simulink model "integer_add_subtract"  (Simulink 7.5)
settings: Solver=ode45  StartTime=0.0  StopTime=10.0  RelTol=1e-3
libraries: xbsIndex_r4 x91
settings Model: Creator=andryc  LastModifiedBy=Murtaza
settings DebuggingCC: StrictBusMsg=Warning

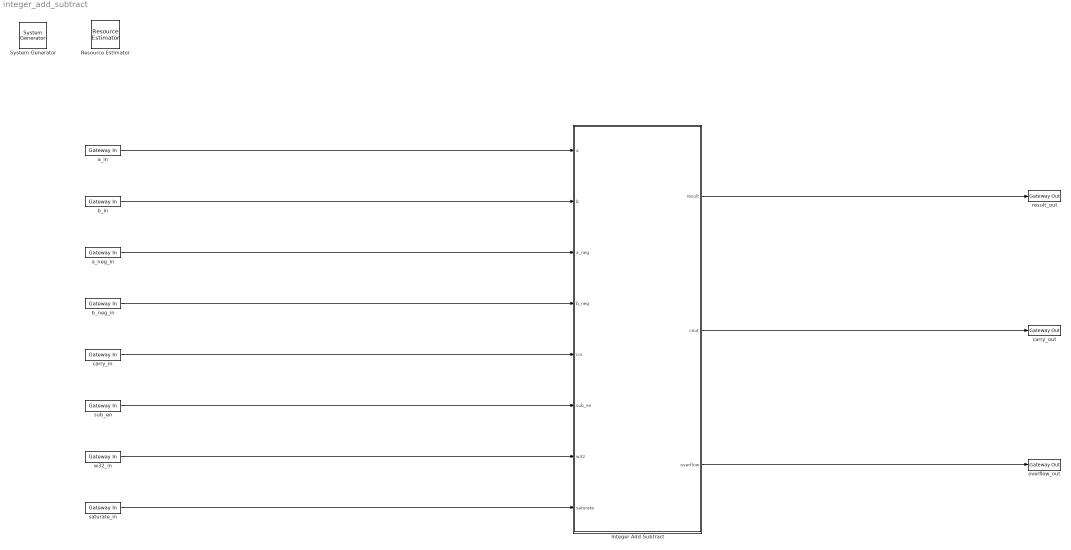
== system integer_add_subtract ==
  " System Generator" : xbsIndex_r4/ System Generator  Tag=genX  SystemSampleTime=-1  xilinxfamily=virtex5  part=xc5vlx330t  speed=-1  package=ff1738  synthesis_tool=XST  clock_wrapper=Clock Enables  directory=./ngc_netlist  proj_type=Project Navigator  testbench=off  simulink_period=1  sysclk_period=3.333333333  dcm_input_clock_period=10  incr_netlist=off  trim_vbits=Everywhere in SubSystem  dbl_ovrd=According to Block Masks  core_generation=According to Block Masks  run_coregen=off  deprecated_control=off  eval_field=0  block_type=sysgen
  Integer Add Subtract : Subsystem
  Resource Estimator : xbsIndex_r4/Resource Estimator  Tag=resEstTag  Slices=0  FFs=0  BRAMs=0  LUTs=0  IOBs=0  EBMs=0  TBUFs=0  xl_use_estimator_area=off  est_options=Estimate  block_type=resource_estimator
      settings: AttributesFormatString=Resource\nEstimator
  a_in : xbsIndex_r4/Gateway In  arith_type=Unsigned  n_bits=32  bin_pt=0  quantization=Truncate  overflow=Saturate  period=1  dbl_ovrd=off  timing_constraint=None  locs_specified=off  LOCs={}  hdl_port=on  block_type=gatewayin
      settings: infoedit="Gateway in block.  Converts inputs of type Simulink integer, double and fixed point to  Xilinx fixed point type.<br><br>Hardware notes:  In hardware these blocks become top level input ports."
  a_neg_in : xbsIndex_r4/Gateway In  arith_type=Unsigned  n_bits=1  bin_pt=0  quantization=Truncate  overflow=Saturate  period=1  dbl_ovrd=off  timing_constraint=None  locs_specified=off  LOCs={}  hdl_port=on  block_type=gatewayin
      settings: infoedit="Gateway in block.  Converts inputs of type Simulink integer, double and fixed point to  Xilinx fixed point type.<br><br>Hardware notes:  In hardware these blocks become top level input ports."
  b_in : xbsIndex_r4/Gateway In  arith_type=Unsigned  n_bits=32  bin_pt=0  quantization=Truncate  overflow=Saturate  period=1  dbl_ovrd=off  timing_constraint=None  locs_specified=off  LOCs={}  hdl_port=on  block_type=gatewayin
      settings: infoedit="Gateway in block.  Converts inputs of type Simulink integer, double and fixed point to  Xilinx fixed point type.<br><br>Hardware notes:  In hardware these blocks become top level input ports."
  b_neg_in : xbsIndex_r4/Gateway In  arith_type=Unsigned  n_bits=1  bin_pt=0  quantization=Truncate  overflow=Saturate  period=1  dbl_ovrd=off  timing_constraint=None  locs_specified=off  LOCs={}  hdl_port=on  block_type=gatewayin
      settings: infoedit="Gateway in block.  Converts inputs of type Simulink integer, double and fixed point to  Xilinx fixed point type.<br><br>Hardware notes:  In hardware these blocks become top level input ports."
  carry_in : xbsIndex_r4/Gateway In  arith_type=Unsigned  n_bits=1  bin_pt=0  quantization=Truncate  overflow=Saturate  period=1  dbl_ovrd=off  timing_constraint=None  locs_specified=off  LOCs={}  hdl_port=on  block_type=gatewayin
      settings: infoedit="Gateway in block.  Converts inputs of type Simulink integer, double and fixed point to  Xilinx fixed point type.<br><br>Hardware notes:  In hardware these blocks become top level input ports."
  carry_out : xbsIndex_r4/Gateway Out  hdl_port=on  timing_constraint=None  locs_specified=off  LOCs={}  block_type=gatewayout
      settings: infoedit="Gateway out block.  Converts Xilinx fixed point inputs into ouputs of type Simulink integer, double, or fixed point.<br><br>Hardware notes:  In hardware these blocks become top level output ports or are discarded, depending on how they are configured."
  overflow_out : xbsIndex_r4/Gateway Out  hdl_port=on  timing_constraint=None  locs_specified=off  LOCs={}  block_type=gatewayout
      settings: infoedit="Gateway out block.  Converts Xilinx fixed point inputs into ouputs of type Simulink integer, double, or fixed point.<br><br>Hardware notes:  In hardware these blocks become top level output ports or are discarded, depending on how they are configured."
  result_out : xbsIndex_r4/Gateway Out  hdl_port=on  timing_constraint=None  locs_specified=off  LOCs={}  block_type=gatewayout
      settings: infoedit="Gateway out block.  Converts Xilinx fixed point inputs into ouputs of type Simulink integer, double, or fixed point.<br><br>Hardware notes:  In hardware these blocks become top level output ports or are discarded, depending on how they are configured."
  saturate_in : xbsIndex_r4/Gateway In  arith_type=Unsigned  n_bits=1  bin_pt=0  quantization=Truncate  overflow=Saturate  period=1  dbl_ovrd=off  timing_constraint=None  locs_specified=off  LOCs={}  hdl_port=on  block_type=gatewayin
      settings: infoedit="Gateway in block.  Converts inputs of type Simulink integer, double and fixed point to  Xilinx fixed point type.<br><br>Hardware notes:  In hardware these blocks become top level input ports."
  sub_en : xbsIndex_r4/Gateway In  arith_type=Unsigned  n_bits=1  bin_pt=0  quantization=Truncate  overflow=Saturate  period=1  dbl_ovrd=off  timing_constraint=None  locs_specified=off  LOCs={}  hdl_port=on  block_type=gatewayin
      settings: infoedit="Gateway in block.  Converts inputs of type Simulink integer, double and fixed point to  Xilinx fixed point type.<br><br>Hardware notes:  In hardware these blocks become top level input ports."
  w32_in : xbsIndex_r4/Gateway In  arith_type=Unsigned  n_bits=1  bin_pt=0  quantization=Truncate  overflow=Saturate  period=1  dbl_ovrd=off  timing_constraint=None  locs_specified=off  LOCs={}  hdl_port=on  block_type=gatewayin
      settings: infoedit="Gateway in block.  Converts inputs of type Simulink integer, double and fixed point to  Xilinx fixed point type.<br><br>Hardware notes:  In hardware these blocks become top level input ports."
  wires:
  a_in/1 -> Integer Add Subtract/1(a)
  b_in/1 -> Integer Add Subtract/2(b)
  a_neg_in/1 -> Integer Add Subtract/3(a_neg)
  b_neg_in/1 -> Integer Add Subtract/4(b_neg)
  carry_in/1 -> Integer Add Subtract/5(cin)
  sub_en/1 -> Integer Add Subtract/6(sub_en)
  w32_in/1 -> Integer Add Subtract/7(w32)
  saturate_in/1 -> Integer Add Subtract/8(saturate)
  Integer Add Subtract/1(result) -> result_out/1
  Integer Add Subtract/2(cout) -> carry_out/1
  Integer Add Subtract/3(overflow) -> overflow_out/1

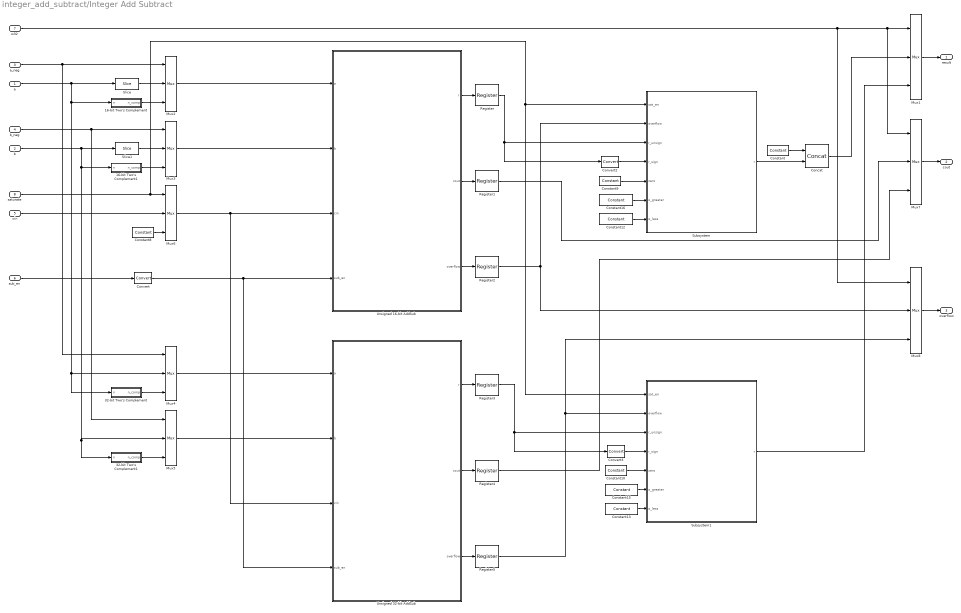
== system integer_add_subtract/Integer Add Subtract ==
  a : Inport
  b : Inport  Port=2
  a_neg : Inport  Port=3
  b_neg : Inport  Port=4
  cin : Inport  Port=5
  sub_en : Inport  Port=6
  w32 : Inport  Port=7
  saturate : Inport  Port=8
  16-bit Two's Complement : Subsystem
  16-bit Two's Complement1 : Subsystem
  32-bit Two's Complement : Subsystem
  32-bit Two's Complement1 : Subsystem
  Concat : xbsIndex_r4/Concat  num_inputs=2  dbl_ovrd=off  block_type=concat
  Constant : xbsIndex_r4/Constant  arith_type=Unsigned  const=0  n_bits=16  bin_pt=0  explicit_period=off  period=1  equ=P=C  opselect=C  inp2=PCIN>>17  opr=+  inp1=P  carry=CIN  dbl_ovrd=off  block_type=constant
  Constant10 : xbsIndex_r4/Constant  arith_type=Signed (2's comp)  const=0  n_bits=32  bin_pt=0  explicit_period=off  period=1  equ=P=C  opselect=C  inp2=PCIN>>17  opr=+  inp1=P  carry=CIN  dbl_ovrd=off  block_type=constant
  Constant12 : xbsIndex_r4/Constant  arith_type=Unsigned  const=32767  n_bits=16  bin_pt=0  explicit_period=off  period=1  equ=P=C  opselect=C  inp2=PCIN>>17  opr=+  inp1=P  carry=CIN  dbl_ovrd=off  block_type=constant
  Constant13 : xbsIndex_r4/Constant  arith_type=Unsigned  const=2147483647  n_bits=32  bin_pt=0  explicit_period=off  period=1  equ=P=C  opselect=C  inp2=PCIN>>17  opr=+  inp1=P  carry=CIN  dbl_ovrd=off  block_type=constant
  Constant15 : xbsIndex_r4/Constant  arith_type=Unsigned  const=2147483648  n_bits=32  bin_pt=0  explicit_period=off  period=1  equ=P=C  opselect=C  inp2=PCIN>>17  opr=+  inp1=P  carry=CIN  dbl_ovrd=off  block_type=constant
  Constant16 : xbsIndex_r4/Constant  arith_type=Unsigned  const=32768  n_bits=16  bin_pt=0  explicit_period=off  period=1  equ=P=C  opselect=C  inp2=PCIN>>17  opr=+  inp1=P  carry=CIN  dbl_ovrd=off  block_type=constant
  Constant8 : xbsIndex_r4/Constant  arith_type=Unsigned  const=0  n_bits=1  bin_pt=0  explicit_period=off  period=1  equ=P=C  opselect=C  inp2=PCIN>>17  opr=+  inp1=P  carry=CIN  dbl_ovrd=off  block_type=constant
  Constant9 : xbsIndex_r4/Constant  arith_type=Signed (2's comp)  const=0  n_bits=16  bin_pt=0  explicit_period=off  period=1  equ=P=C  opselect=C  inp2=PCIN>>17  opr=+  inp1=P  carry=CIN  dbl_ovrd=off  block_type=constant
  Convert : xbsIndex_r4/Convert  arith_type=Boolean  n_bits=16  bin_pt=14  quantization=Truncate  overflow=Wrap  en=off  latency=0  dbl_ovrd=off  pipeline=off  block_type=convert
  Convert2 : xbsIndex_r4/Convert  arith_type="Signed  (2's comp)"  n_bits=16  bin_pt=0  quantization=Truncate  overflow=Saturate  en=off  latency=0  dbl_ovrd=off  pipeline=off  block_type=convert
  Convert3 : xbsIndex_r4/Convert  arith_type="Signed  (2's comp)"  n_bits=32  bin_pt=0  quantization=Truncate  overflow=Saturate  en=off  latency=0  dbl_ovrd=off  pipeline=off  block_type=convert
  Mux{1..8} (8 alike) : xbsIndex_r4/Mux  inputs=2  en=off  latency=0  precision=Full  arith_type=Unsigned  n_bits=16  bin_pt=14  quantization=Truncate  overflow=Wrap  dbl_ovrd=off  block_type=mux
  Register{,1..5} (6 alike) : xbsIndex_r4/Register  init=0  rst=off  en=off  dbl_ovrd=off  block_type=register
  Slice : xbsIndex_r4/Slice  nbits=16  boolean_output=off  mode=Lower Bit Location + Width  bit1=0  base1=MSB of Input  bit0=0  base0=LSB of Input  dbl_ovrd=off  block_type=slice
  Slice1 : xbsIndex_r4/Slice  nbits=16  boolean_output=off  mode=Lower Bit Location + Width  bit1=0  base1=MSB of Input  bit0=0  base0=LSB of Input  dbl_ovrd=off  block_type=slice
  Subsystem : Subsystem
  Subsystem1 : Subsystem
  Unsigned 16-bit AddSub : Subsystem
  Unsigned 32-bit AddSub : Subsystem
  result : Outport
  cout : Outport  Port=2
  overflow : Outport  Port=3
  wires:
  Convert/1 -> Unsigned 32-bit AddSub/4(sub_en), Unsigned 16-bit AddSub/4(sub_en)
  Mux2/1 -> Unsigned 16-bit AddSub/1(a)
  16-bit Two's Complement/1(n_comp) -> Mux2/3
  Slice/1 -> Mux2/2
  Mux3/1 -> Unsigned 16-bit AddSub/2(b)
  Slice1/1 -> Mux3/2
  16-bit Two's Complement1/1(n_comp) -> Mux3/3
  Mux4/1 -> Unsigned 32-bit AddSub/1(a)
  32-bit Two's Complement/1(n_comp) -> Mux4/3
  Mux5/1 -> Unsigned 32-bit AddSub/2(b)
  32-bit Two's Complement1/1(n_comp) -> Mux5/3
  Mux6/1 -> Unsigned 16-bit AddSub/3(cin), Unsigned 32-bit AddSub/3(cin)
  Constant8/1 -> Mux6/3
  Convert2/1 -> Subsystem/4(r_sign)
  Constant9/1 -> Subsystem/5(zero)
  Unsigned 16-bit AddSub/3(overflow) -> Register2/1
  Constant12/1 -> Subsystem/7(o_less)
  Constant16/1 -> Subsystem/6(o_greater)
  Unsigned 16-bit AddSub/1(r) -> Register/1
  Unsigned 32-bit AddSub/3(overflow) -> Register5/1
  Constant10/1 -> Subsystem1/5(zero)
  Convert3/1 -> Subsystem1/4(r_sign)
  Unsigned 32-bit AddSub/1(r) -> Register3/1
  Constant15/1 -> Subsystem1/6(o_greater)
  Constant13/1 -> Subsystem1/7(o_less)
  Subsystem1/1(r) -> Mux1/3
  Mux1/1 -> result/1
  Mux7/1 -> cout/1
  Unsigned 16-bit AddSub/2(cout) -> Register1/1
  Unsigned 32-bit AddSub/2(cout) -> Register4/1
  Mux8/1 -> overflow/1
  w32/1 -> Mux1/1, Mux7/1, Mux8/1
  a_neg/1 -> Mux2/1, Mux4/1
  a/1 -> 16-bit Two's Complement/1(n), 32-bit Two's Complement/1(n), Mux4/2, Slice/1
  b_neg/1 -> Mux3/1, Mux5/1
  b/1 -> 32-bit Two's Complement1/1(n), Mux5/2, 16-bit Two's Complement1/1(n), Slice1/1
  saturate/1 -> Mux6/1, Subsystem/1(sat_en), Subsystem1/1(sat_en)
  cin/1 -> Mux6/2
  sub_en/1 -> Convert/1
  Subsystem/1(r) -> Concat/2
  Concat/1 -> Mux1/2
  Constant/1 -> Concat/1
  Register/1 -> Convert2/1, Subsystem/3(r_unsign)
  Register1/1 -> Mux7/2
  Register2/1 -> Subsystem/2(overflow), Mux8/2
  Register3/1 -> Convert3/1, Subsystem1/3(r_unsign)
  Register4/1 -> Mux7/3
  Register5/1 -> Subsystem1/2(overflow), Mux8/3

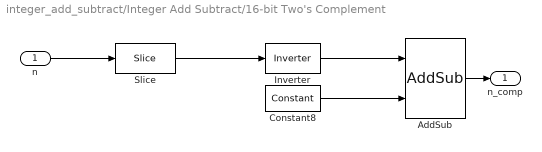
== system integer_add_subtract/Integer Add Subtract/16-bit Two's Complement ==
  n : Inport
  AddSub : xbsIndex_r4/AddSub  mode=Addition  use_carryin=off  use_carryout=off  en=off  latency=0  precision=User Defined  arith_type=Unsigned  n_bits=16  bin_pt=0  quantization=Truncate  overflow=Wrap  dbl_ovrd=off  use_behavioral_HDL=off  hw_selection=Fabric  pipelined=off  block_type=addsub
  Constant8 : xbsIndex_r4/Constant  arith_type=Signed (2's comp)  const=1  n_bits=16  bin_pt=14  explicit_period=off  period=1  equ=P=C  opselect=C  inp2=PCIN>>17  opr=+  inp1=P  carry=CIN  dbl_ovrd=off  block_type=constant
  Inverter : xbsIndex_r4/Inverter  en=off  latency=0  dbl_ovrd=off  block_type=inv
  Slice : xbsIndex_r4/Slice  nbits=16  boolean_output=off  mode=Lower Bit Location + Width  bit1=0  base1=MSB of Input  bit0=0  base0=LSB of Input  dbl_ovrd=off  block_type=slice
  n_comp : Outport
  wires:
  AddSub/1 -> n_comp/1
  n/1 -> Slice/1
  Constant8/1 -> AddSub/2
  Inverter/1 -> AddSub/1
  Slice/1 -> Inverter/1

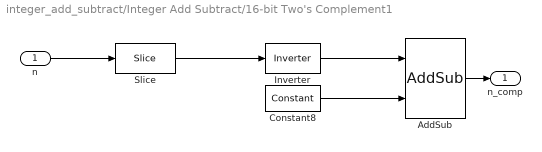
== system integer_add_subtract/Integer Add Subtract/16-bit Two's Complement1 ==
  n : Inport
  AddSub : xbsIndex_r4/AddSub  mode=Addition  use_carryin=off  use_carryout=off  en=off  latency=0  precision=User Defined  arith_type=Unsigned  n_bits=16  bin_pt=0  quantization=Truncate  overflow=Wrap  dbl_ovrd=off  use_behavioral_HDL=off  hw_selection=Fabric  pipelined=off  block_type=addsub
  Constant8 : xbsIndex_r4/Constant  arith_type=Signed (2's comp)  const=1  n_bits=16  bin_pt=14  explicit_period=off  period=1  equ=P=C  opselect=C  inp2=PCIN>>17  opr=+  inp1=P  carry=CIN  dbl_ovrd=off  block_type=constant
  Inverter : xbsIndex_r4/Inverter  en=off  latency=0  dbl_ovrd=off  block_type=inv
  Slice : xbsIndex_r4/Slice  nbits=16  boolean_output=off  mode=Lower Bit Location + Width  bit1=0  base1=MSB of Input  bit0=0  base0=LSB of Input  dbl_ovrd=off  block_type=slice
  n_comp : Outport
  wires:
  Slice/1 -> Inverter/1
  Inverter/1 -> AddSub/1
  Constant8/1 -> AddSub/2
  n/1 -> Slice/1
  AddSub/1 -> n_comp/1

== system integer_add_subtract/Integer Add Subtract/32-bit Two's Complement ==
  n : Inport
  AddSub : xbsIndex_r4/AddSub  mode=Addition  use_carryin=off  use_carryout=off  en=off  latency=0  precision=User Defined  arith_type=Unsigned  n_bits=32  bin_pt=0  quantization=Truncate  overflow=Wrap  dbl_ovrd=off  use_behavioral_HDL=off  hw_selection=Fabric  pipelined=off  block_type=addsub
  Constant8 : xbsIndex_r4/Constant  arith_type=Signed (2's comp)  const=1  n_bits=16  bin_pt=14  explicit_period=off  period=1  equ=P=C  opselect=C  inp2=PCIN>>17  opr=+  inp1=P  carry=CIN  dbl_ovrd=off  block_type=constant
  Inverter : xbsIndex_r4/Inverter  en=off  latency=0  dbl_ovrd=off  block_type=inv
  n_comp : Outport
  wires:
  Inverter/1 -> AddSub/1
  Constant8/1 -> AddSub/2
  n/1 -> Inverter/1
  AddSub/1 -> n_comp/1

== system integer_add_subtract/Integer Add Subtract/32-bit Two's Complement1 ==
  n : Inport
  AddSub : xbsIndex_r4/AddSub  mode=Addition  use_carryin=off  use_carryout=off  en=off  latency=0  precision=User Defined  arith_type=Unsigned  n_bits=32  bin_pt=0  quantization=Truncate  overflow=Wrap  dbl_ovrd=off  use_behavioral_HDL=off  hw_selection=Fabric  pipelined=off  block_type=addsub
  Constant8 : xbsIndex_r4/Constant  arith_type=Signed (2's comp)  const=1  n_bits=16  bin_pt=14  explicit_period=off  period=1  equ=P=C  opselect=C  inp2=PCIN>>17  opr=+  inp1=P  carry=CIN  dbl_ovrd=off  block_type=constant
  Inverter : xbsIndex_r4/Inverter  en=off  latency=0  dbl_ovrd=off  block_type=inv
  n_comp : Outport
  wires:
  AddSub/1 -> n_comp/1
  n/1 -> Inverter/1
  Constant8/1 -> AddSub/2
  Inverter/1 -> AddSub/1

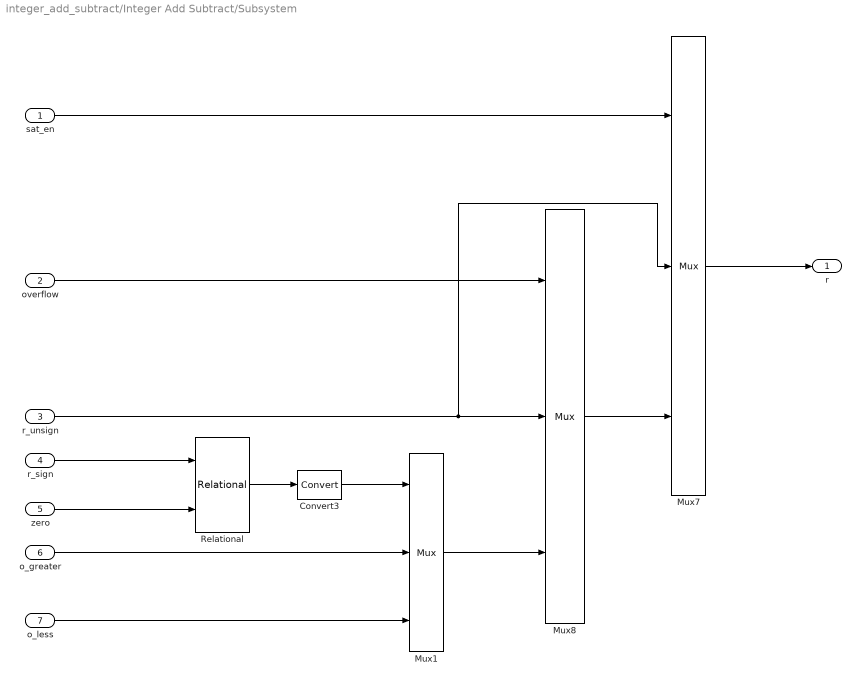
== system integer_add_subtract/Integer Add Subtract/Subsystem ==
  sat_en : Inport
  overflow : Inport  Port=2
  r_unsign : Inport  Port=3
  r_sign : Inport  Port=4
  zero : Inport  Port=5
  o_greater : Inport  Port=6
  o_less : Inport  Port=7
  Convert3 : xbsIndex_r4/Convert  arith_type=Unsigned  n_bits=1  bin_pt=0  quantization=Truncate  overflow=Saturate  en=off  latency=0  dbl_ovrd=off  pipeline=off  block_type=convert
  Mux1 : xbsIndex_r4/Mux  inputs=2  en=off  latency=0  precision=Full  arith_type=Unsigned  n_bits=16  bin_pt=14  quantization=Truncate  overflow=Wrap  dbl_ovrd=off  block_type=mux
  Mux7 : xbsIndex_r4/Mux  inputs=2  en=off  latency=0  precision=Full  arith_type=Unsigned  n_bits=16  bin_pt=14  quantization=Truncate  overflow=Wrap  dbl_ovrd=off  block_type=mux
  Mux8 : xbsIndex_r4/Mux  inputs=2  en=off  latency=0  precision=Full  arith_type=Unsigned  n_bits=16  bin_pt=14  quantization=Truncate  overflow=Wrap  dbl_ovrd=off  block_type=mux
  Relational : xbsIndex_r4/Relational  mode=a<b  en=off  latency=0  dbl_ovrd=off  block_type=relational
  r : Outport
  wires:
  Relational/1 -> Convert3/1
  Convert3/1 -> Mux1/1
  Mux1/1 -> Mux8/3
  Mux8/1 -> Mux7/3
  sat_en/1 -> Mux7/1
  r_unsign/1 -> Mux8/2, Mux7/2
  Mux7/1 -> r/1
  overflow/1 -> Mux8/1
  zero/1 -> Relational/2
  o_greater/1 -> Mux1/2
  o_less/1 -> Mux1/3
  r_sign/1 -> Relational/1

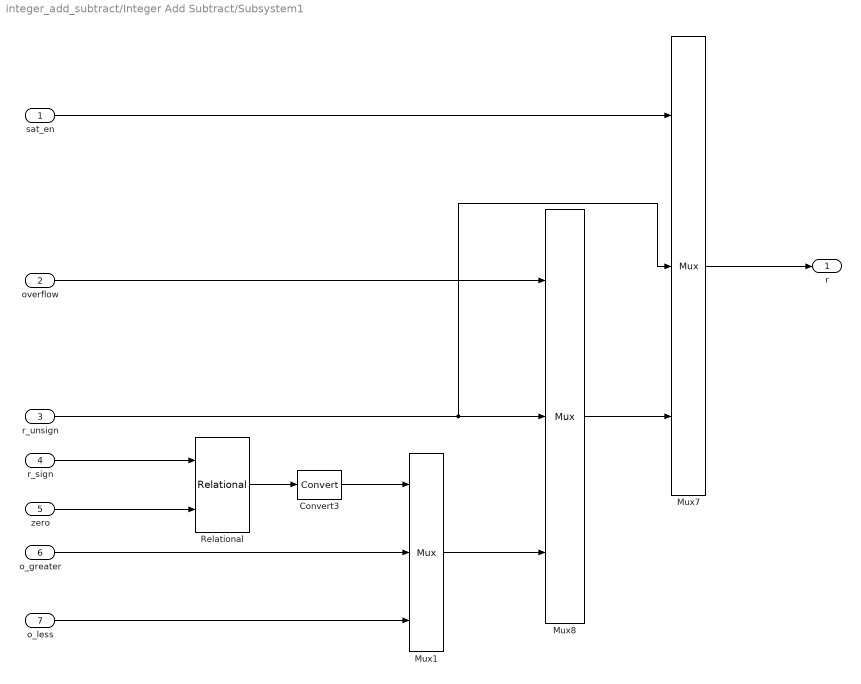
== system integer_add_subtract/Integer Add Subtract/Subsystem1 ==
  sat_en : Inport
  overflow : Inport  Port=2
  r_unsign : Inport  Port=3
  r_sign : Inport  Port=4
  zero : Inport  Port=5
  o_greater : Inport  Port=6
  o_less : Inport  Port=7
  Convert3 : xbsIndex_r4/Convert  arith_type=Unsigned  n_bits=1  bin_pt=0  quantization=Truncate  overflow=Saturate  en=off  latency=0  dbl_ovrd=off  pipeline=off  block_type=convert
  Mux1 : xbsIndex_r4/Mux  inputs=2  en=off  latency=0  precision=Full  arith_type=Unsigned  n_bits=16  bin_pt=14  quantization=Truncate  overflow=Wrap  dbl_ovrd=off  block_type=mux
  Mux7 : xbsIndex_r4/Mux  inputs=2  en=off  latency=0  precision=Full  arith_type=Unsigned  n_bits=16  bin_pt=14  quantization=Truncate  overflow=Wrap  dbl_ovrd=off  block_type=mux
  Mux8 : xbsIndex_r4/Mux  inputs=2  en=off  latency=0  precision=Full  arith_type=Unsigned  n_bits=16  bin_pt=14  quantization=Truncate  overflow=Wrap  dbl_ovrd=off  block_type=mux
  Relational : xbsIndex_r4/Relational  mode=a<b  en=off  latency=0  dbl_ovrd=off  block_type=relational
  r : Outport
  wires:
  r_sign/1 -> Relational/1
  o_less/1 -> Mux1/3
  o_greater/1 -> Mux1/2
  zero/1 -> Relational/2
  overflow/1 -> Mux8/1
  Mux7/1 -> r/1
  r_unsign/1 -> Mux7/2, Mux8/2
  sat_en/1 -> Mux7/1
  Mux8/1 -> Mux7/3
  Mux1/1 -> Mux8/3
  Convert3/1 -> Mux1/1
  Relational/1 -> Convert3/1

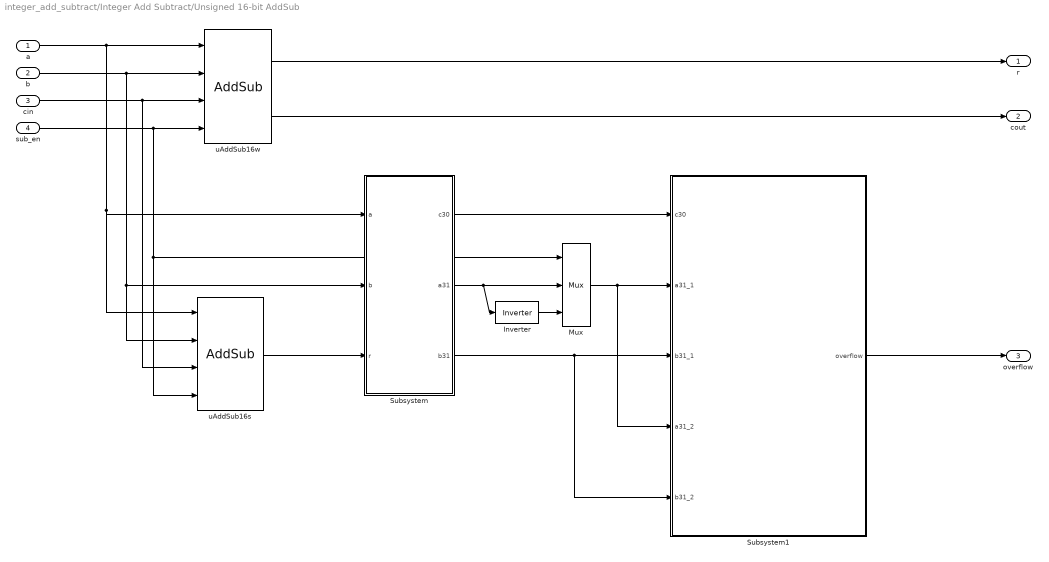
== system integer_add_subtract/Integer Add Subtract/Unsigned 16-bit AddSub ==
  a : Inport
  b : Inport  Port=2
  cin : Inport  Port=3
  sub_en : Inport  Port=4
  Inverter : xbsIndex_r4/Inverter  en=off  latency=0  dbl_ovrd=off  block_type=inv
  Mux : xbsIndex_r4/Mux  inputs=2  en=off  latency=0  precision=Full  arith_type=Unsigned  n_bits=16  bin_pt=14  quantization=Truncate  overflow=Wrap  dbl_ovrd=off  block_type=mux
  Subsystem : Subsystem
  Subsystem1 : Subsystem
  uAddSub16s : xbsIndex_r4/AddSub  mode=Addition or Subtraction  use_carryin=on  use_carryout=off  en=off  latency=0  precision=User Defined  arith_type=Unsigned  n_bits=16  bin_pt=0  quantization=Truncate  overflow=Saturate  dbl_ovrd=off  use_behavioral_HDL=off  hw_selection=Fabric  pipelined=off  block_type=addsub
  uAddSub16w : xbsIndex_r4/AddSub  mode=Addition or Subtraction  use_carryin=on  use_carryout=on  en=off  latency=0  precision=User Defined  arith_type=Unsigned  n_bits=16  bin_pt=0  quantization=Truncate  overflow=Wrap  dbl_ovrd=off  use_behavioral_HDL=off  hw_selection=Fabric  pipelined=off  block_type=addsub
  r : Outport
  cout : Outport  Port=2
  overflow : Outport  Port=3
  wires:
  Inverter/1 -> Mux/3
  Subsystem/2(a31) -> Inverter/1, Mux/2
  Subsystem/3(b31) -> Subsystem1/5(b31_2), Subsystem1/3(b31_1)
  Mux/1 -> Subsystem1/4(a31_2), Subsystem1/2(a31_1)
  Subsystem/1(c30) -> Subsystem1/1(c30)
  uAddSub16w/2 -> cout/1
  Subsystem1/1(overflow) -> overflow/1
  uAddSub16w/1 -> r/1
  sub_en/1 -> uAddSub16w/4, Mux/1, uAddSub16s/4
  cin/1 -> uAddSub16w/3, uAddSub16s/3
  b/1 -> uAddSub16w/2, Subsystem/2(b), uAddSub16s/2
  a/1 -> uAddSub16w/1, Subsystem/1(a), uAddSub16s/1
  uAddSub16s/1 -> Subsystem/3(r)

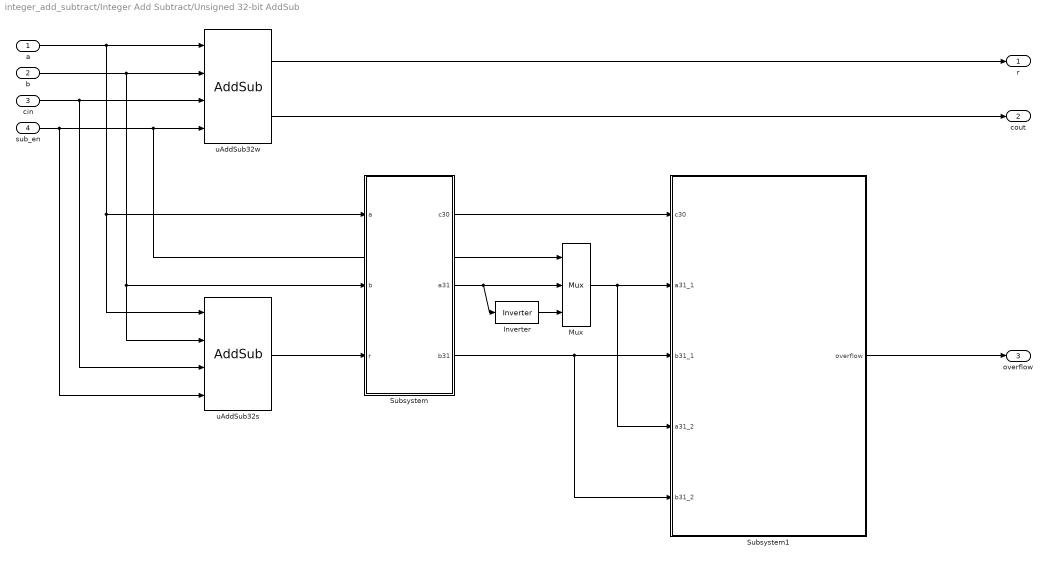
== system integer_add_subtract/Integer Add Subtract/Unsigned 32-bit AddSub ==
  a : Inport
  b : Inport  Port=2
  cin : Inport  Port=3
  sub_en : Inport  Port=4
  Inverter : xbsIndex_r4/Inverter  en=off  latency=0  dbl_ovrd=off  block_type=inv
  Mux : xbsIndex_r4/Mux  inputs=2  en=off  latency=0  precision=Full  arith_type=Unsigned  n_bits=16  bin_pt=14  quantization=Truncate  overflow=Wrap  dbl_ovrd=off  block_type=mux
  Subsystem : Subsystem
  Subsystem1 : Subsystem
  uAddSub32s : xbsIndex_r4/AddSub  mode=Addition or Subtraction  use_carryin=on  use_carryout=off  en=off  latency=0  precision=User Defined  arith_type=Unsigned  n_bits=32  bin_pt=0  quantization=Truncate  overflow=Saturate  dbl_ovrd=off  use_behavioral_HDL=off  hw_selection=Fabric  pipelined=off  block_type=addsub
  uAddSub32w : xbsIndex_r4/AddSub  mode=Addition or Subtraction  use_carryin=on  use_carryout=on  en=off  latency=0  precision=User Defined  arith_type=Unsigned  n_bits=32  bin_pt=0  quantization=Truncate  overflow=Wrap  dbl_ovrd=off  use_behavioral_HDL=off  hw_selection=Fabric  pipelined=off  block_type=addsub
  r : Outport
  cout : Outport  Port=2
  overflow : Outport  Port=3
  wires:
  a/1 -> Subsystem/1(a), uAddSub32s/1, uAddSub32w/1
  b/1 -> Subsystem/2(b), uAddSub32s/2, uAddSub32w/2
  cin/1 -> uAddSub32w/3, uAddSub32s/3
  sub_en/1 -> uAddSub32w/4, Mux/1, uAddSub32s/4
  uAddSub32w/1 -> r/1
  Subsystem1/1(overflow) -> overflow/1
  uAddSub32w/2 -> cout/1
  Subsystem/1(c30) -> Subsystem1/1(c30)
  Mux/1 -> Subsystem1/2(a31_1), Subsystem1/4(a31_2)
  Subsystem/3(b31) -> Subsystem1/3(b31_1), Subsystem1/5(b31_2)
  Subsystem/2(a31) -> Inverter/1, Mux/2
  Inverter/1 -> Mux/3
  uAddSub32s/1 -> Subsystem/3(r)

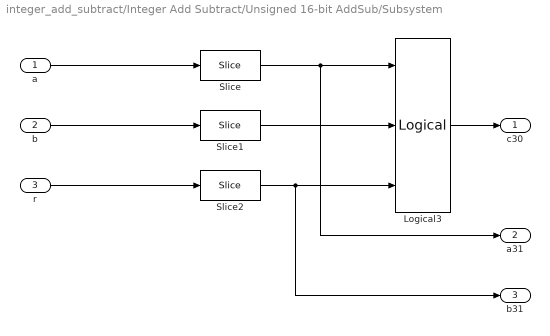
== system integer_add_subtract/Integer Add Subtract/Unsigned 16-bit AddSub/Subsystem ==
  a : Inport
  b : Inport  Port=2
  r : Inport  Port=3
  Logical3 : xbsIndex_r4/Logical  logical_function=XOR  inputs=3  en=off  latency=0  precision=Full  arith_type=Unsigned  n_bits=16  bin_pt=0  align_bp=on  dbl_ovrd=off  block_type=logical
  Slice : xbsIndex_r4/Slice  nbits=1  boolean_output=off  mode=Upper Bit Location + Width  bit1=0  base1=MSB of Input  bit0=0  base0=LSB of Input  dbl_ovrd=off  block_type=slice
  Slice1 : xbsIndex_r4/Slice  nbits=1  boolean_output=off  mode=Upper Bit Location + Width  bit1=0  base1=MSB of Input  bit0=0  base0=LSB of Input  dbl_ovrd=off  block_type=slice
  Slice2 : xbsIndex_r4/Slice  nbits=1  boolean_output=off  mode=Upper Bit Location + Width  bit1=0  base1=MSB of Input  bit0=0  base0=LSB of Input  dbl_ovrd=off  block_type=slice
  c30 : Outport
  a31 : Outport  Port=2
  b31 : Outport  Port=3
  wires:
  Slice2/1 -> b31/1, Logical3/3
  Slice1/1 -> Logical3/2
  Slice/1 -> a31/1, Logical3/1
  Logical3/1 -> c30/1
  r/1 -> Slice2/1
  b/1 -> Slice1/1
  a/1 -> Slice/1

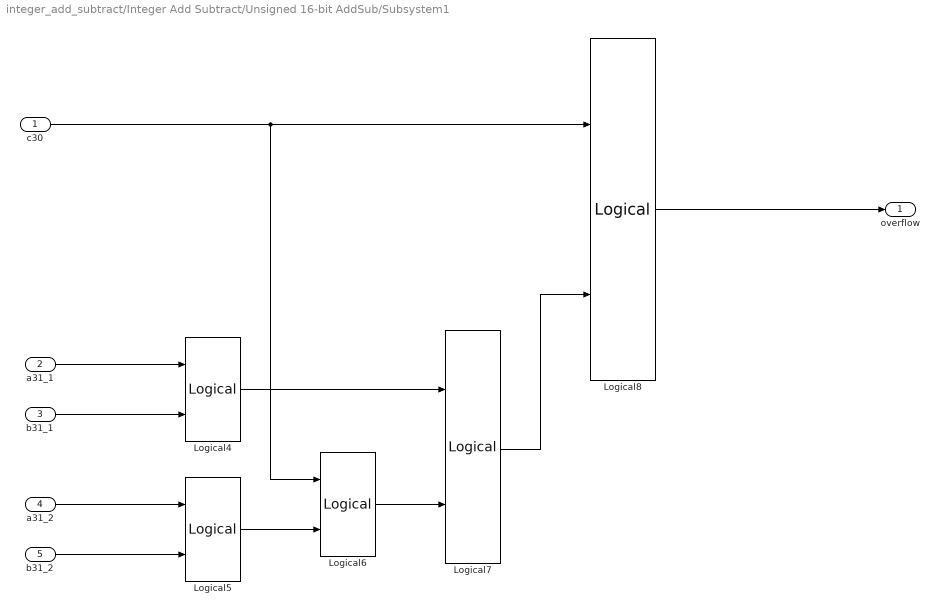
== system integer_add_subtract/Integer Add Subtract/Unsigned 16-bit AddSub/Subsystem1 ==
  c30 : Inport
  a31_1 : Inport  Port=2
  b31_1 : Inport  Port=3
  a31_2 : Inport  Port=4
  b31_2 : Inport  Port=5
  Logical4 : xbsIndex_r4/Logical  logical_function=AND  inputs=2  en=off  latency=0  precision=Full  arith_type=Unsigned  n_bits=16  bin_pt=0  align_bp=on  dbl_ovrd=off  block_type=logical
  Logical5 : xbsIndex_r4/Logical  logical_function=OR  inputs=2  en=off  latency=0  precision=Full  arith_type=Unsigned  n_bits=16  bin_pt=0  align_bp=on  dbl_ovrd=off  block_type=logical
  Logical6 : xbsIndex_r4/Logical  logical_function=AND  inputs=2  en=off  latency=0  precision=Full  arith_type=Unsigned  n_bits=16  bin_pt=0  align_bp=on  dbl_ovrd=off  block_type=logical
  Logical7 : xbsIndex_r4/Logical  logical_function=OR  inputs=2  en=off  latency=0  precision=Full  arith_type=Unsigned  n_bits=16  bin_pt=0  align_bp=on  dbl_ovrd=off  block_type=logical
  Logical8 : xbsIndex_r4/Logical  logical_function=XOR  inputs=2  en=off  latency=0  precision=Full  arith_type=Unsigned  n_bits=16  bin_pt=0  align_bp=on  dbl_ovrd=off  block_type=logical
  overflow : Outport
  wires:
  b31_2/1 -> Logical5/2
  a31_2/1 -> Logical5/1
  b31_1/1 -> Logical4/2
  a31_1/1 -> Logical4/1
  Logical8/1 -> overflow/1
  Logical7/1 -> Logical8/2
  Logical6/1 -> Logical7/2
  Logical4/1 -> Logical7/1
  c30/1 -> Logical6/1, Logical8/1
  Logical5/1 -> Logical6/2

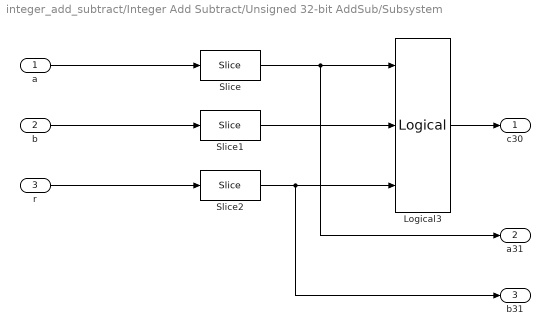
== system integer_add_subtract/Integer Add Subtract/Unsigned 32-bit AddSub/Subsystem ==
  a : Inport
  b : Inport  Port=2
  r : Inport  Port=3
  Logical3 : xbsIndex_r4/Logical  logical_function=XOR  inputs=3  en=off  latency=0  precision=Full  arith_type=Unsigned  n_bits=16  bin_pt=0  align_bp=on  dbl_ovrd=off  block_type=logical
  Slice : xbsIndex_r4/Slice  nbits=1  boolean_output=off  mode=Upper Bit Location + Width  bit1=0  base1=MSB of Input  bit0=0  base0=LSB of Input  dbl_ovrd=off  block_type=slice
  Slice1 : xbsIndex_r4/Slice  nbits=1  boolean_output=off  mode=Upper Bit Location + Width  bit1=0  base1=MSB of Input  bit0=0  base0=LSB of Input  dbl_ovrd=off  block_type=slice
  Slice2 : xbsIndex_r4/Slice  nbits=1  boolean_output=off  mode=Upper Bit Location + Width  bit1=0  base1=MSB of Input  bit0=0  base0=LSB of Input  dbl_ovrd=off  block_type=slice
  c30 : Outport
  a31 : Outport  Port=2
  b31 : Outport  Port=3
  wires:
  a/1 -> Slice/1
  b/1 -> Slice1/1
  r/1 -> Slice2/1
  Logical3/1 -> c30/1
  Slice/1 -> Logical3/1, a31/1
  Slice1/1 -> Logical3/2
  Slice2/1 -> Logical3/3, b31/1

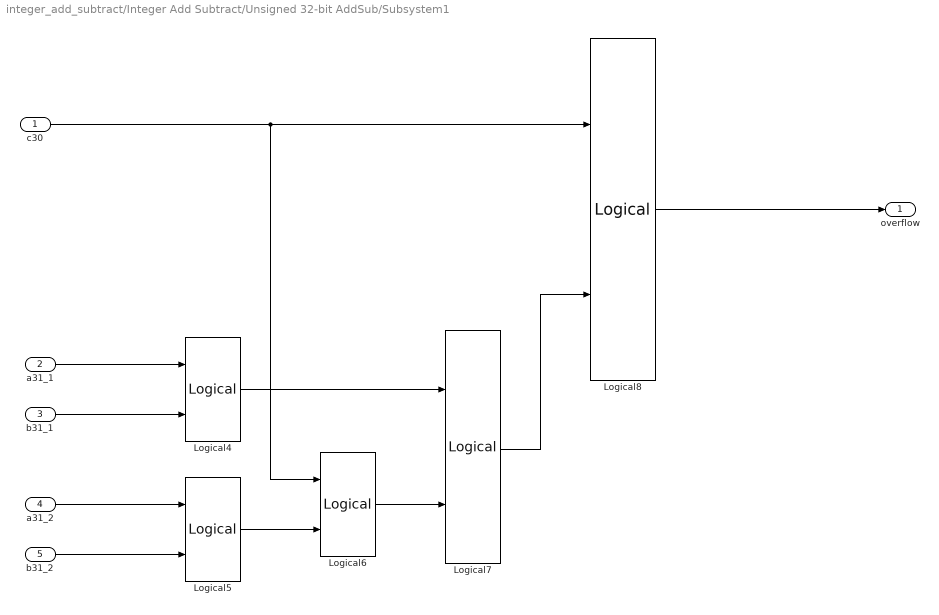
== system integer_add_subtract/Integer Add Subtract/Unsigned 32-bit AddSub/Subsystem1 ==
  c30 : Inport
  a31_1 : Inport  Port=2
  b31_1 : Inport  Port=3
  a31_2 : Inport  Port=4
  b31_2 : Inport  Port=5
  Logical4 : xbsIndex_r4/Logical  logical_function=AND  inputs=2  en=off  latency=0  precision=Full  arith_type=Unsigned  n_bits=16  bin_pt=0  align_bp=on  dbl_ovrd=off  block_type=logical
  Logical5 : xbsIndex_r4/Logical  logical_function=OR  inputs=2  en=off  latency=0  precision=Full  arith_type=Unsigned  n_bits=16  bin_pt=0  align_bp=on  dbl_ovrd=off  block_type=logical
  Logical6 : xbsIndex_r4/Logical  logical_function=AND  inputs=2  en=off  latency=0  precision=Full  arith_type=Unsigned  n_bits=16  bin_pt=0  align_bp=on  dbl_ovrd=off  block_type=logical
  Logical7 : xbsIndex_r4/Logical  logical_function=OR  inputs=2  en=off  latency=0  precision=Full  arith_type=Unsigned  n_bits=16  bin_pt=0  align_bp=on  dbl_ovrd=off  block_type=logical
  Logical8 : xbsIndex_r4/Logical  logical_function=XOR  inputs=2  en=off  latency=0  precision=Full  arith_type=Unsigned  n_bits=16  bin_pt=0  align_bp=on  dbl_ovrd=off  block_type=logical
  overflow : Outport
  wires:
  Logical5/1 -> Logical6/2
  c30/1 -> Logical8/1, Logical6/1
  Logical4/1 -> Logical7/1
  Logical6/1 -> Logical7/2
  Logical7/1 -> Logical8/2
  Logical8/1 -> overflow/1
  a31_1/1 -> Logical4/1
  b31_1/1 -> Logical4/2
  a31_2/1 -> Logical5/1
  b31_2/1 -> Logical5/2
